simulink model "simplePatientModelTuning_01_11_23"  (R2023b)
settings: Solver=VariableStepAuto  StartTime=0.0  StopTime=simTime  FixedStep=0.01  MaxStep=1e-3  RelTol=1e-5
model workspace (MATLAB code in the model file):
  | invState = invState';
values from neighbouring files (symbols this model uses):
  alpha = -1/(cutInValue-15)    (= 0.5)    [simscapeModelParameters_16_08_tuning.m]
  beta = 3.2576    [simscapeModelParameters_16_08_tuning.m]
  breathsTillEE = 3    [simscapeModelParameters_16_08_tuning.m]
  Compliance = 1/13.8    (= 0.0724637681159)    [simscapeModelParameters_16_08_tuning.m]
  Kp = X(1)    [derive_vent_control_param.m]    (also in simscapeModelParameters_16_08_tuning.m = 3)
  lengthEEOcc = 5    [simscapeModelParameters_16_08_tuning.m]
  maxAllowableChange = 5    [simscapeModelParameters_16_08_tuning.m]
  numberOfRecordingsEE = 3    [simscapeModelParameters_16_08_tuning.m]
  Paw_Ref = 11    [simscapeModelParameters_16_08_tuning.m]
  Paw_Threshold = -1    [simscapeModelParameters_16_08_tuning.m]
  PEEP = 5    [simscapeModelParameters_16_08_tuning.m]
  Q_Threshold_Percentage = 0.36    [simscapeModelParameters_16_08_tuning.m]
  Resistance = 8.25    [simscapeModelParameters_16_08_tuning.m]
  Ti = X(2)    [derive_vent_control_param.m]    (also in simscapeModelParameters_16_08_tuning.m = 0.1)
  zeta = 0.3258    [simscapeModelParameters_16_08_tuning.m]
undefined symbols (not defined in the file or in its folder): C_prop_init, C_prop_vector, initial_peak_effort, pmus_array, PS_array
libraries: simulink x1
settings Model: Creator=292636H  LastModifiedBy=292636H

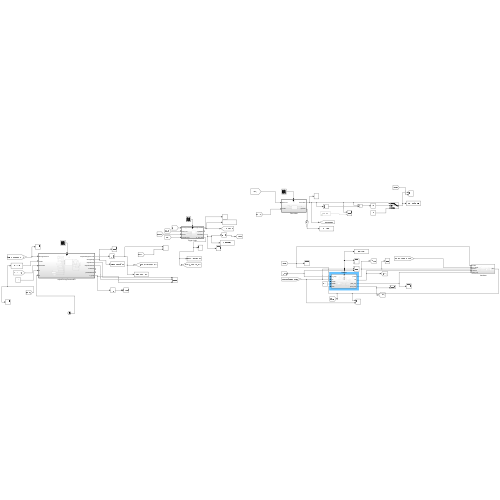
[thumbnail: Simulink's stored preview of the top-level diagram]
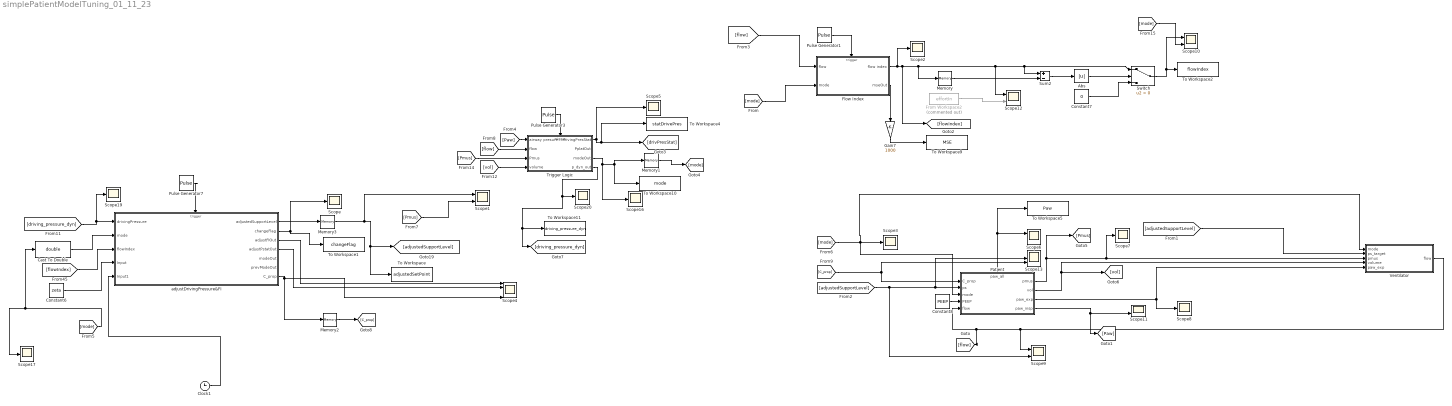
== system simplePatientModelTuning_01_11_23 ==
  Abs : Abs  SaturateOnIntegerOverflow=off
  Cast To Double : DataTypeConversion  OutDataTypeStr=double  SaturateOnIntegerOverflow=off  RndMeth=Floor
  Clock1 : Clock
  Constant6 : Constant  Value=zeta
  Constant7 : Constant  Value=0
  Constant8 : Constant  Value=PEEP
  Flow Index : Subsystem
  From Workspace2 : FromWorkspace  Commented=on  VariableName=effortIn
  Gain7 : Gain  Gain=1000
  Memory : Memory  InheritSampleTime=on
  Memory1 : Memory
  Memory2 : Memory
  Memory3 : Memory
  Patient : Subsystem
      settings: PortSchema="{\"entries\":[{\"content\":{\"sides\":[{\"content\":{\"connectorIds\":[\"In1\",\"In2\",\"In3\",\"In4\",\"In5\"]},\"type\":\"ConnectorPlacement.EquallySpacedRectSide\",\"uuid\":\"07ec80f4-f926-4053-aaff-bfefdf1096b5\"},{\"content\":{\"connectorIds\":[\"Out1\",\"Out2\",\"Out3\",\"Out4\"],\"side\":\"RIGHT\"},\"type\":\"ConnectorPlacement.EquallySpacedRectSide\",\"uuid\":\"ff8c6ed4-5b34-4f3c-9ecb-b1c00a10bd47\"},{\"content\":{\"side\":\"TOP\"},\"type\":\"ConnectorPlacement.EquallySpacedRectSide\",\"uuid\":\"8057a3c4-4a72-4aee-91e9-1f999543c09b\"},{\"content\":{\"connectorIds\":[\"Out5\"],\"side\":\"BOTTOM\"},\"type\":\"ConnectorPlacement.EquallySpacedRectSide\",\"uuid\":\"2e7d54e2-fe50-48e3-a003-97b97c99ab85\"}]},\"type\":\"ConnectorPlacement.EquallySpacedConnector\",\"uuid\":\"fd3741f5-4e20-42f7-9158-5ae2e907869d\"}],\"packageUris\":[\"http://schema.mathworks.com/mf0/Connector/R2020b\"],\"version\":\"1.0\"}"
  Pulse Generator1 : DiscretePulseGenerator  PulseType=Time based  Period=0.01  PulseWidth=5  PhaseDelay=0.01
  Pulse Generator3 : DiscretePulseGenerator  PulseType=Time based  Period=0.01  PulseWidth=5  PhaseDelay=0.01
  Pulse Generator7 : DiscretePulseGenerator  PulseType=Time based  Period=0.01  PulseWidth=5  PhaseDelay=0.01
  Scope{,2..3,5,7..8,16..17,19..20} (10 alike) : Scope
  Scope{1,6,9..12} (6 alike) : Scope  NumInputPorts=2
  Scope13 : Scope  NumInputPorts=3
  Scope4 : Scope  NumInputPorts=4
  Sum2 : Sum  Inputs=+-
  Switch : Switch  Criteria=u2 > Threshold  SaturateOnIntegerOverflow=off  InputSameDT=off
  To Workspace : ToWorkspace  VariableName=adjustedSetPoint  SaveFormat=Timeseries  SampleTime=-1
  To Workspace1 : ToWorkspace  VariableName=changeFlag  SaveFormat=Timeseries  SampleTime=-1
  To Workspace10 : ToWorkspace  VariableName=mode  SaveFormat=Timeseries  SampleTime=-1
  To Workspace11 : ToWorkspace  VariableName=driving_pressure_dyn  SaveFormat=Timeseries  SampleTime=-1
  To Workspace2 : ToWorkspace  VariableName=flowIndex  SaveFormat=Timeseries  SampleTime=-1
  To Workspace4 : ToWorkspace  VariableName=statDrivePres  SaveFormat=Timeseries  SampleTime=-1
  To Workspace5 : ToWorkspace  VariableName=Paw  SaveFormat=Timeseries  SampleTime=-1
  To Workspace9 : ToWorkspace  VariableName=MSE  SaveFormat=Timeseries  SampleTime=-1
  Trigger Logic : Subsystem
  Ventilator : Subsystem
  adjustDrivingPressure&FI : Subsystem  TreatAsAtomicUnit=on
  wires:
  [flow] -> Flow Index/1(flow)
  Pulse Generator1/1 -> Flow Index/Trigger
  Flow Index/1(flow index) -> Scope2/1, [flowIndex], Memory/1, Switch/1, Sum2/1, Scope12/1
  Trigger Logic/1(drivingPresStat) -> To Workspace4/1, [drivPresStat], Scope5/1
  Pulse Generator7/1 -> adjustDrivingPressure&FI/Trigger
  [flowIndex] -> adjustDrivingPressure&FI/3(flowIndex)
  [driving_pressure_dyn] -> Scope19/1, adjustDrivingPressure&FI/1(drivingPressure)
  Constant6/1 -> adjustDrivingPressure&FI/4(Input)
  Pulse Generator3/1 -> Trigger Logic/Trigger
  adjustDrivingPressure&FI/1(adjustedSupportLevel) -> Memory3/1
  Flow Index/2(mseOut) -> Gain7/1
  Clock1/1 -> adjustDrivingPressure&FI/5(Input1)
  [mode] -> Cast To Double/1, Scope17/1
  Cast To Double/1 -> adjustDrivingPressure&FI/2("mode ")
  adjustDrivingPressure&FI/2(changeFlag) -> To Workspace1/1, Scope/1
  adjustDrivingPressure&FI/3(adjustFIOut) -> Scope4/1
  adjustDrivingPressure&FI/4(adjustPstatOut) -> Scope4/2
  Sum2/1 -> Abs/1
  Memory/1 -> Sum2/2
  Abs/1 -> Switch/2
  Constant7/1 -> Switch/3
  Switch/1 -> Scope10/1, To Workspace2/1
  Gain7/1 -> To Workspace9/1
  Trigger Logic/3(modeOut) -> Scope16/1, To Workspace10/1, Memory1/1
  [mode] -> Flow Index/2(mode)
  From Workspace2/1 -> Scope12/2
  [flow] -> Trigger Logic/2(flow)
  [Paw] -> Trigger Logic/1(airway presure)
  [vol] -> Trigger Logic/4(volume)
  [Pmus] -> Trigger Logic/3(Pmus)
  Memory3/1 -> Scope1/1, To Workspace/1, [adjustedSupportLevel]
  [mode] -> Scope10/2
  Trigger Logic/4(p_dyn_out) -> Scope20/1, To Workspace11/1, [driving_pressure_dyn]
  [adjustedSupportLevel] -> Ventilator/2(ps_target)
  Ventilator/1(flow) -> Scope9/1, Patient/1(flow), [flow]
  Patient/3(vol) -> [vol], Ventilator/4(volume)
  [mode] -> Ventilator/1(mode), Scope3/1, Patient/3(mode)
  Patient/5(paw_all) -> Scope6/1, To Workspace5/1
  Constant8/1 -> Patient/2(PEEP)
  Patient/1(paw_insp) -> [Paw], Scope11/2
  Patient/2(paw_exp) -> Ventilator/5(paw_exp), Scope8/1
  [adjustedSupportLevel] -> Scope13/2, Patient/4(ps), Scope9/2
  Patient/4(pmus) -> [Pmus], Scope7/1, Ventilator/3(pmus)
  Memory1/1 -> [mode]
  [Pmus] -> Scope1/2
  adjustDrivingPressure&FI/7(C_prop) -> Memory2/1, Scope4/4
  [C_prop] -> Scope13/3, Patient/5(C_prop)
  Memory2/1 -> [C_prop]

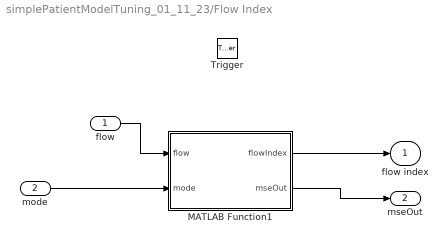
== system simplePatientModelTuning_01_11_23/Flow Index ==
  flow : Inport  LatchByDelayingOutsideSignal=on
  mode : Inport  Port=2
  Trigger : TriggerPort  VariantControl=Variant  PortDimensions=1
  MATLAB Function1 : MATLAB Function  TreatAsAtomicUnit=on
  flow index : Outport
  mseOut : Outport  Port=2
  wires:
  flow/1 -> MATLAB Function1/1(flow)
  MATLAB Function1/1(flowIndex) -> flow index/1
  mode/1 -> MATLAB Function1/2(mode)
  MATLAB Function1/2(mseOut) -> mseOut/1

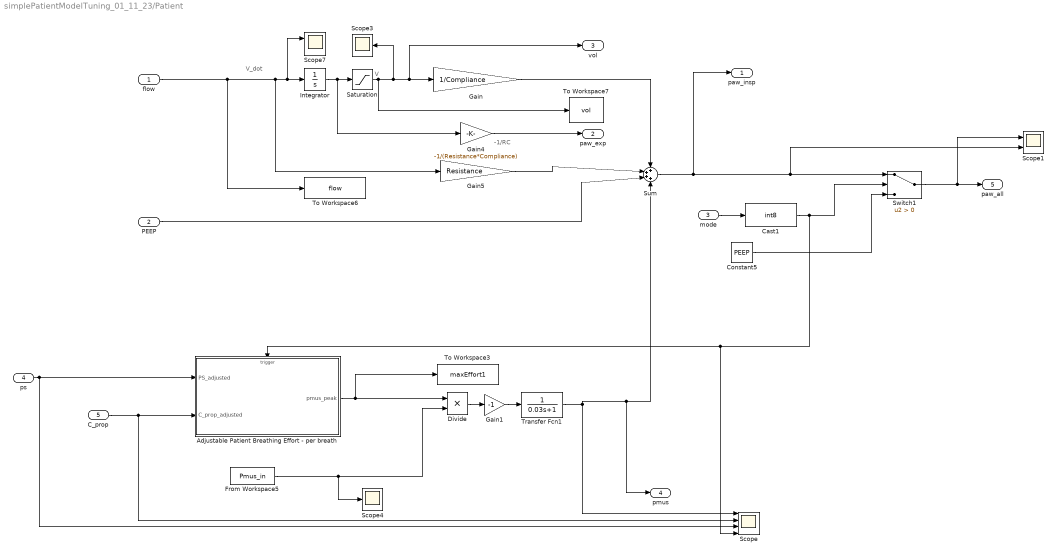
== system simplePatientModelTuning_01_11_23/Patient ==
  note: V
  note: -1/RC
  note: V_dot
  flow : Inport
  PEEP : Inport  Port=2
  mode : Inport  Port=3
  ps : Inport  Port=4
  C_prop : Inport  Port=5
  Adjustable Patient Breathing Effort - per breath : Subsystem
  Cast1 : DataTypeConversion  OutDataTypeStr=int8  SaturateOnIntegerOverflow=off  RndMeth=Floor
  Constant5 : Constant  Value=PEEP
  Divide : Product  Inputs=**
  From Workspace5 : FromWorkspace  VariableName=Pmus_in
  Gain : Gain  Gain=1/Compliance
  Gain1 : Gain  Gain=-1
  Gain4 : Gain  Gain=-1/(Resistance*Compliance)
  Gain5 : Gain  Gain=Resistance
  Integrator : Integrator
  Saturation : Saturate  UpperLimit=10000000  LowerLimit=0
  Scope : Scope  NumInputPorts=4
  Scope1 : Scope  NumInputPorts=2
  Scope3 : Scope
  Scope4 : Scope
  Scope7 : Scope  NumInputPorts=2
  Sum : Sum  Inputs=++++
  Switch1 : Switch  Criteria=u2 > Threshold  SaturateOnIntegerOverflow=off  InputSameDT=off
  To Workspace3 : ToWorkspace  VariableName=maxEffort1  SaveFormat=Timeseries  SampleTime=-1
  To Workspace6 : ToWorkspace  VariableName=flow  SaveFormat=Timeseries  SampleTime=-1
  To Workspace7 : ToWorkspace  VariableName=vol  SaveFormat=Timeseries  SampleTime=-1
  Transfer Fcn1 : TransferFcn  Denominator=[0.03 1]
  paw_insp : Outport
  paw_exp : Outport  Port=2
  vol : Outport  Port=3
  pmus : Outport  Port=4
  paw_all : Outport  Port=5
  wires:
  Saturation/1 -> To Workspace7/1, Scope3/1, vol/1, Gain/1
  Gain4/1 -> paw_exp/1
  flow/1 -> Gain5/1, Scope7/1, Integrator/1, To Workspace6/1
  Integrator/1 -> Gain4/1, Saturation/1
  Gain/1 -> Sum/1
  Gain5/1 -> Sum/2
  PEEP/1 -> Sum/3
  Switch1/1 -> Scope1/1, paw_all/1
  Cast1/1 -> Scope/4, Adjustable Patient Breathing Effort - per breath/Trigger, Switch1/2
  Sum/1 -> Scope1/2, Switch1/1, paw_insp/1
  Constant5/1 -> Switch1/3
  From Workspace5/1 -> Scope4/1, Divide/2
  mode/1 -> Cast1/1
  C_prop/1 -> Scope/2, Adjustable Patient Breathing Effort - per breath/2(C_prop_adjusted)
  Transfer Fcn1/1 -> pmus/1, Sum/4, Scope/1
  Adjustable Patient Breathing Effort - per breath/1(pmus_peak) -> Divide/1, To Workspace3/1
  ps/1 -> Scope/3, Adjustable Patient Breathing Effort - per breath/1(PS_adjusted)
  Divide/1 -> Gain1/1
  Gain1/1 -> Transfer Fcn1/1

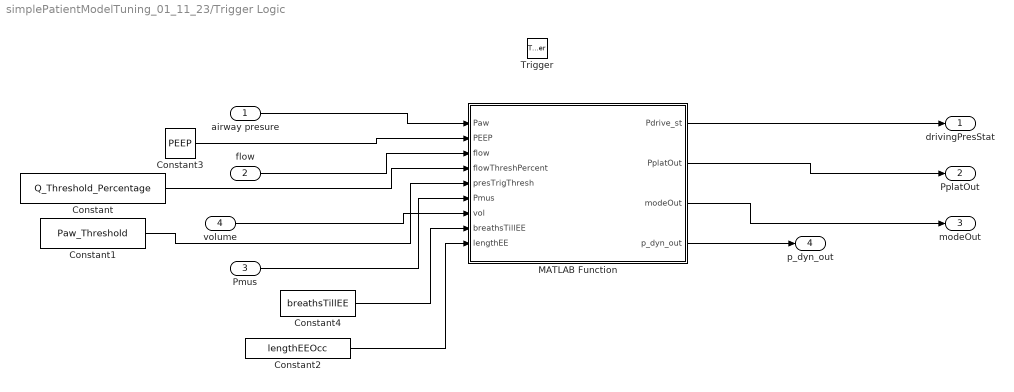
== system simplePatientModelTuning_01_11_23/Trigger Logic ==
  airway presure : Inport  LatchByDelayingOutsideSignal=on
  flow : Inport  Port=2  LatchByDelayingOutsideSignal=on
  Pmus : Inport  Port=3
  volume : Inport  Port=4  LatchByDelayingOutsideSignal=on
  Trigger : TriggerPort  VariantControl=Variant  PortDimensions=1
  Constant : Constant  Value=Q_Threshold_Percentage
  Constant1 : Constant  Value=Paw_Threshold
  Constant2 : Constant  Value=lengthEEOcc
  Constant3 : Constant  Value=PEEP
  Constant4 : Constant  Value=breathsTillEE
  MATLAB Function : MATLAB Function  TreatAsAtomicUnit=on
  drivingPresStat : Outport
  PplatOut : Outport  Port=2
  modeOut : Outport  Port=3
  p_dyn_out : Outport  Port=4
  wires:
  airway presure/1 -> MATLAB Function/1(Paw)
  Constant3/1 -> MATLAB Function/2(PEEP)
  flow/1 -> MATLAB Function/3(flow)
  MATLAB Function/1(Pdrive_st) -> drivingPresStat/1
  MATLAB Function/2(PplatOut) -> PplatOut/1
  Constant/1 -> MATLAB Function/4(flowThreshPercent)
  Constant1/1 -> MATLAB Function/5(presTrigThresh)
  MATLAB Function/3(modeOut) -> modeOut/1
  Pmus/1 -> MATLAB Function/6(Pmus)
  volume/1 -> MATLAB Function/7(vol)
  Constant2/1 -> MATLAB Function/9(lengthEE)
  Constant4/1 -> MATLAB Function/8(breathsTillEE)
  MATLAB Function/4(p_dyn_out) -> p_dyn_out/1

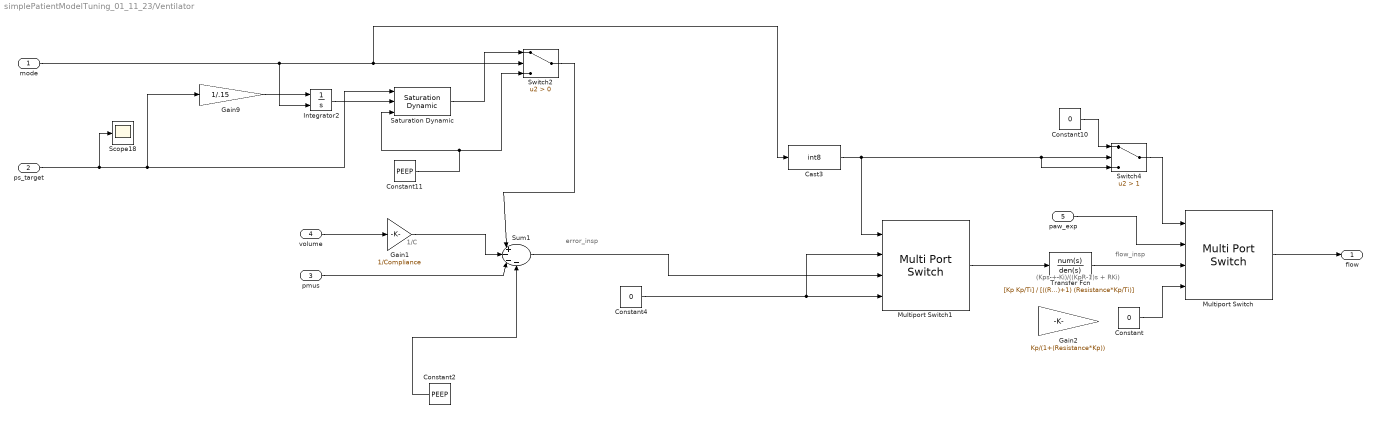
== system simplePatientModelTuning_01_11_23/Ventilator ==
  note: error_insp
  note: 1/C
  note: flow_insp
  note: (Kps + Ki)/((KpR-1)s + RKi)
  mode : Inport
  ps_target : Inport  Port=2
  pmus : Inport  Port=3
  volume : Inport  Port=4
  paw_exp : Inport  Port=5
  Cast3 : DataTypeConversion  OutDataTypeStr=int8  SaturateOnIntegerOverflow=off  RndMeth=Floor
  Constant : Constant  Value=0
  Constant10 : Constant  Value=0
  Constant11 : Constant  Value=PEEP
  Constant2 : Constant  Value=PEEP
  Constant4 : Constant  Value=0
  Gain1 : Gain  Gain=1/Compliance
  Gain2 : Gain  Gain=Kp/(1+(Resistance*Kp))
  Gain9 : Gain  Gain=1/.15
  Integrator2 : Integrator  ExternalReset=rising  InitialCondition=PEEP
  Multiport Switch : MultiPortSwitch  DataPortOrder=Specify indices  DataPortIndices={0,1,2}  SaturateOnIntegerOverflow=off  InputSameDT=off
  Multiport Switch1 : MultiPortSwitch  DataPortOrder=Specify indices  DataPortIndices={0,1,2}  SaturateOnIntegerOverflow=off  InputSameDT=off
  Saturation Dynamic : simulink/Discontinuities/Saturation Dynamic  OutMin=[]  OutMax=[]  OutDataTypeStr=Inherit: Same as second input  OutDataType=fixdt(1, 16)  OutScaling=2^-10  DoSatur=off
  Scope18 : Scope
  Sum1 : Sum  Inputs=|+---
  Switch2 : Switch  Criteria=u2 > Threshold  SaturateOnIntegerOverflow=off  InputSameDT=off
  Switch4 : Switch  Criteria=u2 > Threshold  Threshold=1  SaturateOnIntegerOverflow=off  InputSameDT=off
  Transfer Fcn : TransferFcn  Numerator=[Kp Kp/Ti]  Denominator=[((Resistance*Kp)+1) (Resistance*Kp/Ti)]
  flow : Outport
  wires:
  Constant2/1 -> Sum1/4
  volume/1 -> Gain1/1
  Gain1/1 -> Sum1/2
  pmus/1 -> Sum1/3
  Gain9/1 -> Integrator2/1
  Integrator2/1 -> Saturation Dynamic/2
  ps_target/1 -> Scope18/1, Saturation Dynamic/1, Gain9/1
  Saturation Dynamic/1 -> Switch2/1
  Constant11/1 -> Switch2/3, Saturation Dynamic/3
  Switch2/1 -> Sum1/1
  Sum1/1 -> Multiport Switch1/3
  mode/1 -> Integrator2/2, Cast3/1, Switch2/2
  Constant4/1 -> Multiport Switch1/2, Multiport Switch1/4
  Switch4/1 -> Multiport Switch/1
  Constant10/1 -> Switch4/1
  Cast3/1 -> Switch4/3, Switch4/2, Multiport Switch1/1
  Transfer Fcn/1 -> Multiport Switch/3
  Constant/1 -> Multiport Switch/4
  paw_exp/1 -> Multiport Switch/2
  Multiport Switch/1 -> flow/1
  Multiport Switch1/1 -> Transfer Fcn/1

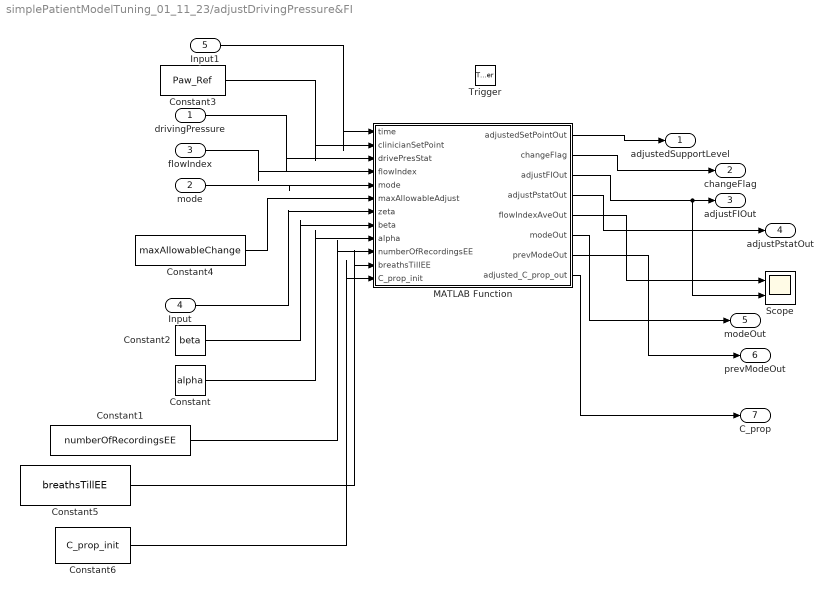
== system simplePatientModelTuning_01_11_23/adjustDrivingPressure&FI ==
  drivingPressure : Inport
  "mode " : Inport  Port=2
  flowIndex : Inport  Port=3
  Input : Inport  Port=4
  Input1 : Inport  Port=5
  Trigger : TriggerPort  VariantControl=Variant
  Constant : Constant  Value=alpha
  Constant1 : Constant  Value=numberOfRecordingsEE
  Constant2 : Constant  Value=beta
  Constant3 : Constant  Value=Paw_Ref
  Constant4 : Constant  Value=maxAllowableChange
  Constant5 : Constant  Value=breathsTillEE
  Constant6 : Constant  Value=C_prop_init
  MATLAB Function : MATLAB Function  TreatAsAtomicUnit=on
  Scope : Scope  NumInputPorts=2
  adjustedSupportLevel : Outport
  changeFlag : Outport  Port=2
  adjustFIOut : Outport  Port=3
  adjustPstatOut : Outport  Port=4
  modeOut : Outport  Port=5
  prevModeOut : Outport  Port=6
  C_prop : Outport  Port=7
  wires:
  MATLAB Function/1(adjustedSetPointOut) -> adjustedSupportLevel/1
  Constant3/1 -> MATLAB Function/2(clinicianSetPoint)
  drivingPressure/1 -> MATLAB Function/3(drivePresStat)
  Constant4/1 -> MATLAB Function/6(maxAllowableAdjust)
  "mode "/1 -> MATLAB Function/5(mode)
  flowIndex/1 -> MATLAB Function/4(flowIndex)
  Constant/1 -> MATLAB Function/9(alpha)
  Input/1 -> MATLAB Function/7(zeta)
  Constant2/1 -> MATLAB Function/8(beta)
  MATLAB Function/2(changeFlag) -> changeFlag/1
  MATLAB Function/3(adjustFIOut) -> Scope/2, adjustFIOut/1
  MATLAB Function/4(adjustPstatOut) -> adjustPstatOut/1
  Input1/1 -> MATLAB Function/1(time)
  MATLAB Function/6(modeOut) -> modeOut/1
  MATLAB Function/7(prevModeOut) -> prevModeOut/1
  MATLAB Function/5(flowIndexAveOut) -> Scope/1
  Constant1/1 -> MATLAB Function/10(numberOfRecordingsEE)
  Constant5/1 -> MATLAB Function/11(breathsTillEE)
  Constant6/1 -> MATLAB Function/12(C_prop_init)
  MATLAB Function/8(adjusted_C_prop_out) -> C_prop/1

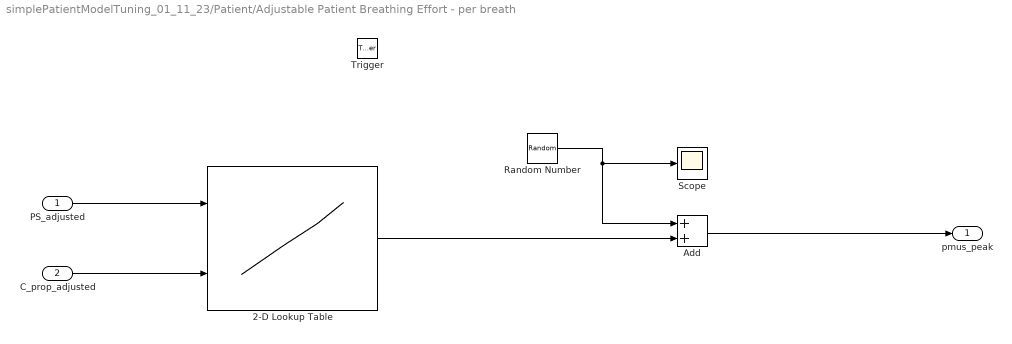
== system simplePatientModelTuning_01_11_23/Patient/Adjustable Patient Breathing Effort - per breath ==
  PS_adjusted : Inport
  C_prop_adjusted : Inport  Port=2
  Trigger : TriggerPort  VariantControl=(inherit)  ShowOutputPort=on  PortDimensions=1
  2-D Lookup Table : Lookup_n-D  BreakpointsForDimension1=C_prop_vector  BreakpointsForDimension2=PS_array  Table=pmus_array  InternalRulePriority=Speed  RndMeth=Simplest
      settings: InputPortMap=u0,u1
  Add : Sum
  Random Number : RandomNumber  Variance=1.56/2
  Scope : Scope
  pmus_peak : Outport  InitialOutput=initial_peak_effort
  wires:
  PS_adjusted/1 -> 2-D Lookup Table/1
  C_prop_adjusted/1 -> 2-D Lookup Table/2
  Random Number/1 -> Add/1, Scope/1
  2-D Lookup Table/1 -> Add/2
  Add/1 -> pmus_peak/1

== matlab function simplePatientModelTuning_01_11_23/Trigger Logic/MATLAB Function ==
  data: Paw input; PEEP input; flow input; Pdrive_st output; PplatOut output; flowThreshPercent input; presTrigThresh input; modeOut output; Pmus input; vol input; breathsTillEE input; lengthEE input; p_dyn_out output
function [Pdrive_st, PplatOut, modeOut, p_dyn_out]  = triggerLogic(Paw,PEEP,flow,...
    flowThreshPercent,presTrigThresh,Pmus,vol,breathsTillEE,lengthEE)

%PERSISTENT VARIABLE DECLERATION
persistent PstCalc; %persistent variable for static driving pressure
persistent Pplat; %plateau pressure
persistent prevMode;
persistent flag;
persistent mode;
persistent peakFlow;
persistent newBreath;
persistent breathCounter1;
persistent x;
persistent pmus_calc;
persistent t;
persistent flag_EE;
persistent paw_peak;
persistent p_dyn_est;

%PERSISTENT VARIABLE DECLERATIONS
if isempty(flag) %initialise ke = 0
    Pplat = 0;
    PstCalc = 0;
    flag = 0;
    prevMode = 0;
    mode = 0;
    peakFlow = 0;
    newBreath = 0;
    breathCounter1 = 0;
    x = 0;
    pmus_calc = PEEP;
    t = 0;
    flag_EE = 0;
    paw_peak = 0;
    p_dyn_est = 0;
end

  %Change Modes
     %change to end-expiratory mode after set number of breaths
 if breathCounter1 == breathsTillEE && mode == 0
      flag_EE= 1;
 end

switch(mode)
    %Expiration
    case 0 %expiration mode
        
        %Reset Counters and variables
        x = 0; %reset breath counter associated variable

        if Pmus > -0.01
            newBreath = 1;
        end
        %Pressure trigger
        PawDiff = Paw - PEEP;
        if PawDiff < presTrigThresh && newBreath == 1
            newBreath = 0;
            if flag_EE == 1
                mode = 2;
            else
                mode = 1; %set state to inspiration
            end 
        end

    %Inspiration
    case 1 %inspiration mode
        
        %count the number of breaths
        if x == 0 %execute only once each breath at start of expiration
            breathCounter1 = breathCounter1 + 1; %increment each breath
            x = 1; %prevent counter from incrementing till next breath
        end
        %%PEAK FLOW
        %Check for cycling off, determine peak flow
        if flow > peakFlow %check for greater flow magnitude than previous
            peakFlow = flow; %set current flow to peak flow
        end

        %DETERMINE CYCLING OFF THRESHOLD FLOW
        threshFlow = peakFlow * flowThreshPercent; %calc cycling off flow

        %cycle off once threshold reached
        if flow < threshFlow %flow dropped below threshold value
            mode = 0; %change to expiration state
            peakFlow = 0; %reset peak flow value
        end

        %%PEAK Pressure
        if Paw > paw_peak
            paw_peak = Paw;
        end
end

%Occlusion record plateau pressure
if mode == 2
    t = t+1;
    if Paw < pmus_calc
        pmus_calc = Paw;
    end

     if t > (lengthEE * 100) %after x seconds has passed      
                %calculate dynamic driving pressure
                pmus_est = (PEEP - pmus_calc);% * 0.75;
                p_dyn_est =  paw_peak - PEEP + 2/3*pmus_est; %calc and store value of Pmus
                
                %reset variables
                pmus_calc = PEEP;
                breathCounter1 = 0; %reset breath counter
                t = 0; %reset timer
                mode = 0; %change back to expiration mode
                flag_EE = 0;
                paw_peak = 0;
     end 
   
end

%Determine static driving pressure after occlusion finishes
if mode == 0 && cast(prevMode, "uint8") == 2
    if flag == 0
	    PstCalc = Pplat - PEEP;
	    Pplat = 0;
        flag = 1;
    end
end
%save previous mode value
if mode ~= prevMode
    prevMode = mode;
end

%output
Pdrive_st = PstCalc;
PplatOut = Pplat;
modeOut = mode;
p_dyn_out = p_dyn_est;
end

== matlab function simplePatientModelTuning_01_11_23/Flow Index/MATLAB Function1 ==
  data: flow input; flowIndex output; mode input; mseOut output
%This function determines the flow index for each breath. The function
%inputs the state and flow signal; and outputs the flow index. During
%inspiration, The magnitude of the flow signal at discrete points in time
%are stored into an array. During expiration, this array is then
%manipulated to obtain a measure of the flow index for the previous
%inspiration. A fitting function is used to obtain the parameters of the
%flow index model, Q(t) = a-b *(change in time)^c

function [flowIndex, mseOut]  = fcn(flow, mode)%, funNonLin)
coder.extrinsic('nonLinFit');
coder.extrinsic('cond_func');
persistent flowMeasured;
persistent x;
persistent k;
persistent i; %counter to check if start of inspiration
persistent e; %counter to check if start of expiration
persistent start; %flag for start of model runtime
persistent c_est_2; %variable to calculate flow index
persistent occFlag; %flag, avoid calculating FI after an occlusion
persistent killSwitch; %exist while loop
%persistent r2Curr; %current R squared value
%persistent QmaxCurr; %current max flow
%accurate flow index
%persistent r2Best; %best fitting determined
persistent c;
persistent c1;
persistent MSE;

%INITIALISE PERSISTENT VARIABLES
if isempty(flowMeasured)
    flowMeasured = zeros(1,1000) -10;
    x = 0;
    k = 1;
    i = 0;
    e = 0;
    start = 1;
    c_est_2 = 0;
    c = 0;
    occFlag = 0;
    c = 0;
    c1 = 0;
    MSE = 0;
    killSwitch = 0;
end

QmaxCurr = 0;


%CHECK FOR OCCLUSIONS
%occlusion modes, signal flag to not determine FI after an occlusion
if mode == 2 || mode == 3
    occFlag = 1; %Set occlusion flag, flow index not determined
end

%reset occFlag during inspiration
if mode == 1
    occFlag = 0; %reset occlusion flag, resume determining flow index
end



%INSPIRATION STATE, RECORD FLOW SIGNAL
if mode == 1 %if in inspiration state

    %check if at start of simulation, wait until first breath to begin
    %recording flow data
    if start == 1
        start = 0;
    end

    %Reset counters from expiration phase
    x = 0; %reset counter that clears other counters during expiration
    e = 0; %reset counter that checks if at start of expiration phase


    %array cell equal to current magnitude of flow
    flowMeasured(1,k) = flow; %store current measure of flow
    %increment array cell counter for each time function block executed
    k = k+1;

end

%EXPIRATION STATE, CALCULATE FLOW INDEX
if mode == 0 %if in expiration state

    %Perform fitting only once per expiration
    if e == 0 && occFlag ~= 1 && start == 0

        time = [0:0.01:(length(flowMeasured)-1)*0.01];


        %DETERMINE INITIAL CUT OFF POINT
        %find where flow increase by more than 1% of proceeding value
        i = 2; %loop variable
        int_ind = 1; %default value, start from first inspiration value recorded

        %loop through entire flow signal array until cut off point
        %determined
        while i < length(flowMeasured) && killSwitch == 0
            %determine difference between 2 subsequent flow readings
            onePercentCheck = ...
                (flowMeasured(i) - flowMeasured(i-1))/flowMeasured(i-1);

            %check if flow rate has increased by more than one percent
            if onePercentCheck < 0.05 && onePercentCheck > 0
                int_ind = i; %save index value
                killSwitch = 1; %set killswitch to exit the loop
            end
            i = i +1; %increment loop variable
        end
            
        [~,int_ind_a] = max(flowMeasured);
        if int_ind_a < int_ind
            int_ind = int_ind_a;
        end
        if int_ind == 1
            [~,int_ind] = max(flowMeasured);
        end

        %DETERMINE END OF RECORDING
        %Determine last index of array where value != -10
        end_ind = find(flowMeasured>-10,1,'last') - 1;

        %create flow array between max flow and last value measured
        flow_array=flowMeasured(int_ind:end_ind(1,1));

        time1 = time(int_ind:end_ind(1,1));

        %DETERMINE CUT OFF POINT
        i = 2; %looping variable
        killSwitch1 = 0; %variable to exit loop early
        cutOffInd = length(flow_array); %if no cut off index determined,
        %maintain current length of array
        %loop through entire flow array
        while i < length(flow_array) && killSwitch1 == 0
            %determine percentage decrease in flow between two
            %measurements
            percentDecrease = (flow_array(i)- flow_array(i-1))/...
                flow_array(i-1);

            %if flow decreases by more than 10%
            if percentDecrease < -0.1
                cutOffInd = i; %save curr index as cut off index value
                killSwitch1 = 1; %set killswitch to exit loop
            end

            i = i + 1; %
        end

        %*********DETERMINE INITIAL ESTIMATES LINEAR FITTING***********
        %create final flow array
        flowFitting = flow_array(1:cutOffInd);
        flowFittingNL = flowFitting;
        timeFitting = time1(1:cutOffInd);
        timeFittingNL = timeFitting;



        %PEAK FLOW
        %find max flow value by taking mean of first 10 values recorded
        %Qmax=mean(flow_array(1:10));
            r2Best = 0;
            flowRateDecrease = 0;
            flowIndexBest = 0;
            QmaxBest = 0;

        if ~isempty(flowFitting)
            [Qmax,maxInd] = max(flowFitting);
            flowFitting= flowFitting(maxInd:end);
            deltaT = timeFitting(maxInd:end);

            if Qmax ~= 0
                for k = 1:1:2
                    for i=0:1:10

                        if k == 1
                            QmaxCurr = Qmax + (0.005*i);
                        end
                        if k == 2
                            QmaxCurr = Qmax - (0.005*i);
                        end

                        deltaQ = QmaxCurr - flowFitting;

                        %FORMAT DATA
                        %remove negative data
                        deltaQFit=deltaQ(find(deltaQ>0));
                        deltaTFit=deltaT(find(deltaQ>0));
                        W = diag(deltaTFit);

                        %take logs of input and output data
                        y=log(deltaQFit);
                        x=log(deltaTFit);

                        %remove -inf/inf values
                        x = x(find(isinf(x) == 0));
                        y = y(find(isinf(x) == 0));

                        %store oupput and input data in matrix form
                        A=[x' ones(size(x'))];
                        B=[y'];

                        %LINEAR LEAST SQUARES ESTIMATION
                        %solve the weighted least sqaure estimation problem to obtain
                        %estimates of decrease in flow rate and flow index
                        %fitting_param_2=inv(A'*W*A)*A'*W*B;
                        fitting_param_2=inv(A'*A)*A'*B;

                        %determine fitting parameter for flow index
                        c_est_2=fitting_param_2(1);
                        b_est_2=-exp(fitting_param_2(2));

                        Q_est_2=Qmax+b_est_2*deltaT.^c_est_2;

                        %determine R2 value
                        r = flowFitting-Q_est_2;
                        normr = norm(r);
                        SSE = normr.^2; %sum of regression
                        %sum of squares
                        SST = norm(flowFitting-mean(flowFitting))^2;
                        R2 = 1 - SSE/SST;
                        r2Curr = R2;

                        %if current fitting is better than all previous
                        %store model parameters
                        if r2Curr > r2Best
                            flowIndexBest = c_est_2;
                            r2Best = r2Curr;
                            flowRateDecrease = b_est_2;
                            QmaxBest = QmaxCurr;
                        end

                    end
                end
            end
        end

        %%%%%%%%%%%%%%%%%%%%%NON LIN FIT%%%%%%%%%%%%%%%%%%%%%%%%%%%%

        beta0 = [QmaxBest,flowRateDecrease,flowIndexBest]; %initial estimates
        X = timeFittingNL; %input data, time
        Y = flowFittingNL; %output data

        beta = zeros(1,3); %declare output variable
        if ~isempty(Y) && ~isempty(X)
            [beta,MSE,flag_ill_cond] = nonLinFit(X,Y,beta0); %perform non-linear fitting
            % beta(2)
            % if beta(2) < -100
            %     beta = [NaN,NaN,NaN];
            %     MSE = NaN;
            % end
            %check if ill-conditioned
           % s = svd(J);
            %cond_j = s(1) / s(3);  % Rough condition number estimate
            %rcond_j = rcond(J);
            % flag_ill_cond_int = int8(flag_ill_cond);
            % if flag_ill_cond_int == 1
            %     beta = [NaN,NaN,NaN];
            %     MSE = NaN;
            % end
        else
            beta = [NaN,NaN,NaN];
            MSE = NaN;
        end

        if ~isnan(beta(3))
            c1 = beta(3);
        else
            c1 = c1;
        end
        %
        plot(X,Y)
        hold on
        plot(X,beta(1)+beta(2).*X.^beta(3))
        hold off
       
    end


    %RESET COUNTERS/VARIABLES
    k = 1; %reset array increment counter
    flowMeasured = zeros(1,1000) -10;
    killSwitch = 0;

    e = e +1;

end

%FUNCTION OUTPUT
flowIndex = c1;
%flowIndexNL = 0; %dummy value
mseOut = MSE;

end

== matlab function simplePatientModelTuning_01_11_23/adjustDrivingPressure&FI/MATLAB Function ==
  data: time input; clinicianSetPoint input; adjustedSetPointOut output; drivePresStat input; flowIndex input; mode input; maxAllowableAdjust input; zeta input; beta input; alpha input; changeFlag output; adjustFIOut output; adjustPstatOut output; flowIndexAveOut output; modeOut output; prevModeOut output; numberOfRecordingsEE input; breathsTillEE input; C_prop_init input; adjusted_C_prop_out output
function [adjustedSetPointOut, changeFlag,adjustFIOut,adjustPstatOut, flowIndexAveOut, modeOut, prevModeOut, adjusted_C_prop_out] = ...
    fcn(time, clinicianSetPoint, drivePresStat,flowIndex,mode,maxAllowableAdjust,...
      zeta, beta, alpha, numberOfRecordingsEE, breathsTillEE, C_prop_init)
    
    %PERSISTENT VARIABLE DECLERATION
    persistent adjustedSetPoint; %change in pressure support
    persistent flowIndexArray; %array store most recent FI values
    persistent adjustPstat; %adjustment due to driving pressure
    persistent adjustFI; %adjustment due to flow index
    persistent adjustTotal; %adjustment accounting for FI and Pstat
    persistent setPointStart; %starting clinician set pressure support value
    persistent prevMode; %store values of previous mode
    persistent flag; %flag to only adjust set point once per occlusion
    persistent prevModeArray;
    persistent flowIndexAve;
    persistent breath_counter;
    persistent flag_breath;
    persistent occ_counter; 
    persistent p_dyn_array;
    persistent adjusted_C_prop;


    %INITIALISE PERSISTENT VARIABLES  
    if isempty(adjustPstat)
        adjustPstat = 0;
        adjustedSetPoint = clinicianSetPoint;
        flowIndexArray = zeros(breathsTillEE*numberOfRecordingsEE,1); %store most recent FI values
        adjustFI = 0;
        adjustTotal = 0;
        setPointStart = clinicianSetPoint;
        prevMode = 0;
        prevModeArray = zeros(5,1);
        flag = 1;
        flowIndexAve = 0;
        breath_counter = 0;
        flag_breath = 1;
        occ_counter = 0;
        p_dyn_array = zeros(numberOfRecordingsEE,1);
        adjusted_C_prop = C_prop_init; 
    end

    changeFlag = 0;

    if mode == 2.2737e-11
        mode = 0;
    end

    if prevMode == 2.2737e-11
        prevMode = 0;
    end

    %%RECORD FLOW INDEX VAUES
    %Record flow index value at the start of new inspiration
    if mode == 0 && prevMode == 1 && flowIndex ~= 0
        flowIndexArray(1) = flowIndex;
        flowIndexArray = circshift(flowIndexArray,1);
        breath_counter = breath_counter + 1; %increment each breath
    end
    
    %Reset flag when end inspiratory occlusion occurs
    if mode == 2 && cast(prevMode, "uint8") == 0
        flag = 0;
    end  
    
    %if 3 occlusions have been preformed take the averages and adjust PS
    if mode == 0 && (cast(prevMode, "uint8") == 2)% || ismember(2,prevModeArray)) 

        occ_counter = occ_counter + 1;
        p_dyn_array(occ_counter) = drivePresStat;

        if occ_counter == 3
        %if mode == 0 && breath_counter >= 5
            %remove 0 values from flow index array
            if flowIndexArray(1) == 0
                flowIndexArrayIP = flowIndexArray(2:end,1);
            else
                flowIndexArrayIP = flowIndexArray;
            end
        
            if flowIndexArrayIP(end) == 0
                endInd = find(flowIndexArrayIP == 0, 1, 'first');
                flowIndexArrayIP = flowIndexArrayIP(1:endInd(1,1)-1);
            end
        
            %FLOW INDEX
            %determine parameters of linear realtionship for function f_1(FI_ave)
            % m = (maxAllowableAdjust - (-maxAllowableAdjust))/(4.5-2.5);
            % c = maxAllowableAdjust - (m*4.5);
            m = (1 - (-1))/(4.5-2.5);
            c = 1 - (m*4.5);
            %determine average
            flowIndexAve = mean(flowIndexArrayIP);
            if flowIndexAve > 4 || flowIndexAve < 3
                adjustFI = m*flowIndexAve + c;
                adjustFI = adjustFI * zeta;
            else
                adjustFI = 0;
            end
            %DRIVING PRESSURE
        
            %introduce saturation limit (curve does not behave as intended where
            %static driving pressure >= 15
            drivPresStatIP = min(14.99,mean(p_dyn_array));
        
            adjustPstat = min((alpha + 1/(drivPresStatIP-15)),0);
       
            %saturation limit
            %adjustPstat = min(maxAllowableAdjust,adjustPstat);
            adjustPstat = adjustPstat * beta;
        
            %ADJUST SET POINT
            adjustTotal = adjustFI + adjustPstat;
            adjustedSetPoint = adjustedSetPoint + adjustTotal;
              
            lowerLimit = setPointStart - maxAllowableAdjust;
            upperLimit = setPointStart + maxAllowableAdjust;
        
            %Apply limits
            adjustedSetPoint = max(lowerLimit,adjustedSetPoint);
            adjustedSetPoint = min(upperLimit,adjustedSetPoint);
        
            %% Adjust Sedation
            
            adjustPstat_sedation = max(-1*(alpha + 1/(drivPresStatIP-15)),0);
            adjusted_C_prop = adjusted_C_prop + adjustPstat_sedation;
            
            %limits
            lower_limit_sedation = 0;
            upper_limit_sedation = 2;

            %Apply limits
            adjusted_C_prop= max(lower_limit_sedation,adjusted_C_prop);
            adjusted_C_prop = min(upper_limit_sedation,adjusted_C_prop);

            %reset variables
            % flowIndexArray = zeros(3,1);
            
            %prevent algorithm from adjusting set point again until next
            %occlusion
            flag = 1;
            changeFlag = 1;
            breath_counter = 0;
            occ_counter = 0;
            p_dyn_array = zeros(numberOfRecordingsEE,1);
        end
    end
    
    %Store previous mode
    prevMode = mode;

    for k=2:length(prevModeArray)
        prevModeArray(k)=prevModeArray(k-1);
    end
    prevModeArray(1)=mode;
    
    %adjustedSetPointOut = adjustedSetPoint;
    adjustedSetPointOut = adjustedSetPoint;
    adjusted_C_prop_out = adjusted_C_prop;
    adjustFIOut = adjustFI;
    adjustPstatOut = adjustPstat;
    flowIndexAveOut = flowIndexAve;
    modeOut = mode;
    prevModeOut = prevMode;
end
